simulink model "sys_ctrl_obs_luenberger_lineal_int_theta"  (Simulink 8.6)
settings: Solver=ode45  StartTime=0.0  StopTime=Tt  RelTol=1e-3
undefined symbols (not defined in the file): A11, A12, A21, A22, Ad, B1, B2, Bd, Cd, Dd, K, Knoise, L, r, Ts, x_0
settings Model: Creator=pdoren  LastModifiedBy=pdoren
settings SolverCC: ZeroCrossAlgorithm=Adaptive
settings DataIOCC: SaveFormat=StructureWithTime  SignalLoggingSaveFormat=Dataset
settings OptimizationCC: ExpressionDepthLimit=128
settings DebuggingCC: UnderspecifiedInitializationDetection=Simplified  MergeDetectMultiDrivingBlocksExec=error  SolverPrmCheckMsg=none  FcnCallInpInsideContextMsg=EnableAllAsWarning  StateNameClashWarn=none
settings HardwareCC: ProdBitPerPointer=64  ProdLargestAtomicFloat=Float  ProdIntDivRoundTo=Zero  ProdEndianess=LittleEndian  ProdHWDeviceType=Specified
settings GRTTargetCC: GeneratePreprocessorConditionals=Use local settings
settings ConfigComp: CovModelRefEnable=off

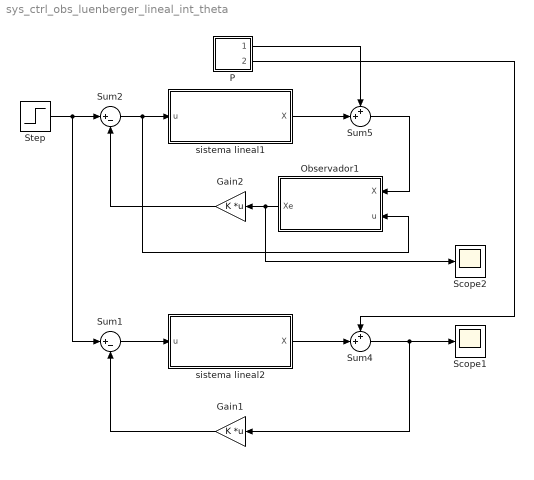
== system sys_ctrl_obs_luenberger_lineal_int_theta ==
  Gain1 : Gain  Gain=K  Multiplication=Matrix(K*u)
  Gain2 : Gain  Gain=K  Multiplication=Matrix(K*u)
  Observador1 : Subsystem
  P : Subsystem
  Scope1 : Scope
  Scope2 : Scope
  Step : Step  After=r  SampleTime=0
  Sum1 : Sum  Inputs=|+-
  Sum2 : Sum  Inputs=|+-
  Sum4 : Sum  Inputs=++|
  Sum5 : Sum  Inputs=++|
  sistema lineal1 : Subsystem
  sistema lineal2 : Subsystem
  wires:
  Sum2/1 -> Observador1/2(u), sistema lineal1/1(u)
  Gain2/1 -> Sum2/2
  sistema lineal1/1(X) -> Sum5/2
  Sum5/1 -> Observador1/1(X)
  Step/1 -> Sum1/1, Sum2/1
  Sum1/1 -> sistema lineal2/1(u)
  Gain1/1 -> Sum1/2
  sistema lineal2/1(X) -> Sum4/2
  Sum4/1 -> Gain1/1, Scope1/1
  P/2(Noise5) -> Sum4/1
  P/1(Noise3) -> Sum5/1
  Observador1/1(Xe) -> Gain2/1, Scope2/1

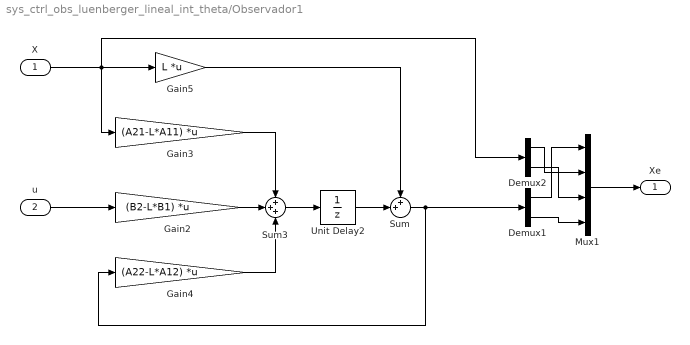
== system sys_ctrl_obs_luenberger_lineal_int_theta/Observador1 ==
  X : Inport
  u : Inport  Port=2
  Demux1 : Demux  Outputs=2
  Demux2 : Demux  Outputs=2
  Gain2 : Gain  Gain=(B2-L*B1)  Multiplication=Matrix(K*u)
  Gain3 : Gain  Gain=(A21-L*A11)  Multiplication=Matrix(K*u)
  Gain4 : Gain  Gain=(A22-L*A12)  Multiplication=Matrix(K*u)
  Gain5 : Gain  Gain=L  Multiplication=Matrix(K*u)
  Mux1 : Mux
  Sum : Sum  Inputs=++|
  Sum3 : Sum  Inputs=+++
  Unit Delay2 : UnitDelay  SampleTime=Ts
  Xe : Outport
  wires:
  Gain3/1 -> Sum3/1
  Gain4/1 -> Sum3/3
  Unit Delay2/1 -> Sum/2
  Sum3/1 -> Unit Delay2/1
  Gain2/1 -> Sum3/2
  Mux1/1 -> Xe/1
  u/1 -> Gain2/1
  Sum/1 -> Gain4/1, Demux1/1
  Gain5/1 -> Sum/1
  X/1 -> Gain3/1, Demux2/1, Gain5/1
  Demux2/2 -> Mux1/3
  Demux2/1 -> Mux1/2
  Demux1/1 -> Mux1/1
  Demux1/2 -> Mux1/4

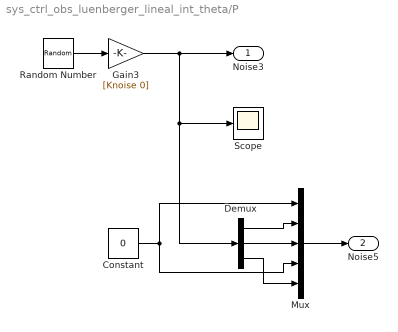
== system sys_ctrl_obs_luenberger_lineal_int_theta/P ==
  Constant : Constant  Value=0
  Demux : Demux  Outputs=3
  Gain3 : Gain  Gain=[Knoise 0]
  Mux : Mux  Inputs=5
  Random Number : RandomNumber  SampleTime=Ts
  Scope : Scope
  Noise3 : Outport
  Noise5 : Outport  Port=2
  wires:
  Random Number/1 -> Gain3/1
  Gain3/1 -> Noise3/1, Demux/1, Scope/1
  Mux/1 -> Noise5/1
  Demux/1 -> Mux/2
  Demux/2 -> Mux/3
  Constant/1 -> Mux/4, Mux/1
  Demux/3 -> Mux/5

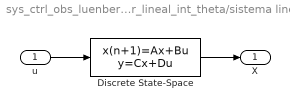
== system sys_ctrl_obs_luenberger_lineal_int_theta/sistema lineal1 ==
  u : Inport
  Discrete State-Space : DiscreteStateSpace  A=Ad  B=Bd  C=Cd  D=Dd  X0=x_0  SampleTime=Ts
  X : Outport
  wires:
  u/1 -> Discrete State-Space/1
  Discrete State-Space/1 -> X/1

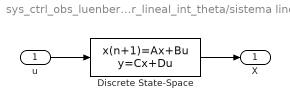
== system sys_ctrl_obs_luenberger_lineal_int_theta/sistema lineal2 ==
  u : Inport
  Discrete State-Space : DiscreteStateSpace  A=Ad  B=Bd  C=eye(5)  D=zeros(5,1)  X0=x_0  SampleTime=Ts
  X : Outport
  wires:
  u/1 -> Discrete State-Space/1
  Discrete State-Space/1 -> X/1
